simulink model "testfx"  (Simulink 6.0)
settings: Solver=ode45  StartTime=0.0  StopTime=10.0  RelTol=1e-3
InitFcn:
  | ;
StartFcn:
  | ;
StopFcn:
  | ;
undefined symbols (not defined in the file or in its folder): dden, tsamp
libraries: simulink x8
PreSaveFcn:
  | ;
CloseFcn:
  | rtwprivate ssgencode ModelCloseRequest testfx;
settings Model: Creator=myunt  LastModifiedBy=myunt  ExtModeAutoUpdateStatusClock=off
settings DebuggingCC: CheckExecutionContextPreStartOutputMsg=on  CheckExecutionContextRuntimeOutputMsg=on

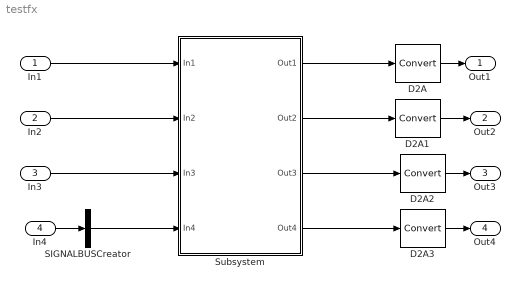
== system testfx ==
  In1 : Inport  LatchInput=off
  In2 : Inport  Port=2  LatchInput=off
  In3 : Inport  Port=3  LatchInput=off
  In4 : Inport  Port=4  LatchInput=off
  D2A{,1..3} (4 alike) : DataTypeConversion  OutDataTypeMode=double
  SIGNALBUSCreator : BusCreator  DialogController=Simulink.DDGSource_Bus  Inputs=1
  Subsystem : Subsystem  TreatAsAtomicUnit=on  PropExecContextAcrossSSBoundary=on
  Out1 : Outport
  Out2 : Outport  Port=2
  Out3 : Outport  Port=3
  Out4 : Outport  Port=4
  wires:
  In1/1 -> Subsystem/1(In1)
  Subsystem/1(Out1) -> D2A/1
  D2A/1 -> Out1/1
  Subsystem/2(Out2) -> D2A1/1
  D2A1/1 -> Out2/1
  In3/1 -> Subsystem/3(In3)
  Subsystem/3(Out3) -> D2A2/1
  D2A2/1 -> Out3/1
  Subsystem/4(Out4) -> D2A3/1
  D2A3/1 -> Out4/1
  In2/1 -> Subsystem/2(In2)
  In4/1 -> SIGNALBUSCreator/1
  SIGNALBUSCreator/1 -> Subsystem/4(In4)

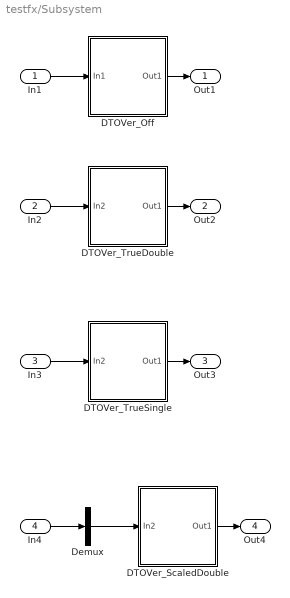
== system testfx/Subsystem ==
  In1 : Inport  LatchInput=off
  In2 : Inport  Port=2  LatchInput=off
  In3 : Inport  Port=3  LatchInput=off
  In4 : Inport  Port=4  LatchInput=off
  DTOVer_Off : Subsystem  PropExecContextAcrossSSBoundary=on
  DTOVer_ScaledDouble : Subsystem  PropExecContextAcrossSSBoundary=on  DataTypeOverride=ScaledDoubles
  DTOVer_TrueDouble : Subsystem  PropExecContextAcrossSSBoundary=on  DataTypeOverride=TrueDoubles
  DTOVer_TrueSingle : Subsystem  PropExecContextAcrossSSBoundary=on  DataTypeOverride=TrueSingles
  Demux : Demux  Outputs=1
  Out1 : Outport
  Out2 : Outport  Port=2
  Out3 : Outport  Port=3
  Out4 : Outport  Port=4
  wires:
  In1/1 -> DTOVer_Off/1(In1)
  DTOVer_Off/1(Out1) -> Out1/1
  In2/1 -> DTOVer_TrueDouble/1(In2)
  DTOVer_TrueDouble/1(Out1) -> Out2/1
  In3/1 -> DTOVer_TrueSingle/1(In2)
  DTOVer_TrueSingle/1(Out1) -> Out3/1
  In4/1 -> Demux/1
  Demux/1 -> DTOVer_ScaledDouble/1(In2)
  DTOVer_ScaledDouble/1(Out1) -> Out4/1

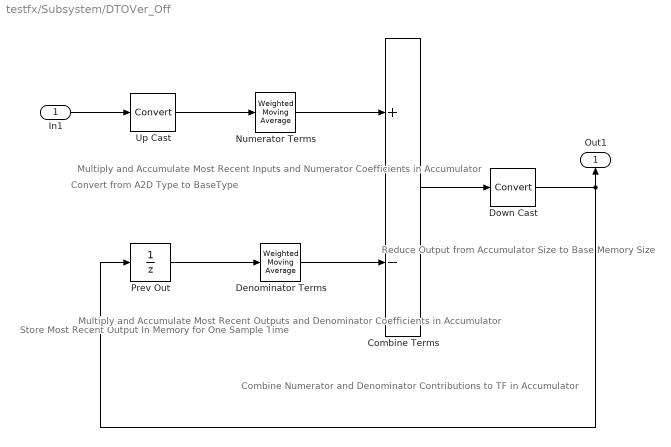
== system testfx/Subsystem/DTOVer_Off ==
  note: Reduce Output from
      | Accumulator Size to
      | Base Memory Size
  note: Combine Numerator
      | and Denominator
      | Contributions to TF
      | in Accumulator
  note: Store Most
      | Recent Output
      | In Memory for
      | One Sample Time
  note: Multiply and Accumulate
      | Most Recent Outputs and
      | Denominator Coefficients
      | in Accumulator
  note: Multiply and Accumulate
      | Most Recent Inputs and
      | Numerator Coefficients
      | in Accumulator
  note: Convert from
      | A2D Type
      | to BaseType
  In1 : Inport  DataType=Specify via dialog  OutScaling=2^-8  LatchInput=off
  Combine Terms : Sum  Inputs=+-  OutDataTypeMode=Specify via dialog  OutDataType=AccumType  OutScaling=2^(-12)  SaturateOnIntegerOverflow=on
  Denominator Terms : simulink/Discrete/Weighted Moving Average  mgainval=dden(2:length(dden))  vinit=0.0  samptime=tsamp  GainDataTypeScalingMode=Specify via dialog  GainDataType=BaseType  MatRadixGroup=Best Precision: Element-wise  GainScaling=2^-14  OutputDataTypeScalingMode=Specify via dialog  OutDataType=AccumType  OutScaling=2^(-12)  DoSatur=on
  Down Cast : DataTypeConversion  OutDataTypeMode=Specify via dialog  OutDataType=BaseType  OutScaling=2^(-5)  SaturateOnIntegerOverflow=on
  Numerator Terms : simulink/Discrete/Weighted Moving Average  mgainval=dnum  vinit=0.0  samptime=tsamp  GainDataTypeScalingMode=Specify via dialog  GainDataType=BaseType  MatRadixGroup=Best Precision: Element-wise  GainScaling=2^-14  OutputDataTypeScalingMode=Specify via dialog  OutDataType=AccumType  OutScaling=2^(-12)  DoSatur=on
  Prev Out : UnitDelay  X0=0.0  SampleTime=tsamp
  Up Cast : DataTypeConversion  OutDataTypeMode=Specify via dialog  OutDataType=BaseType  OutScaling=2^(-14)  SaturateOnIntegerOverflow=on
  Out1 : Outport  Orientation=up  InitialOutput=0
  wires:
  Down Cast/1 -> Out1/1, Prev Out/1
  In1/1 -> Up Cast/1
  Up Cast/1 -> Numerator Terms/1
  Prev Out/1 -> Denominator Terms/1
  Numerator Terms/1 -> Combine Terms/1
  Denominator Terms/1 -> Combine Terms/2
  Combine Terms/1 -> Down Cast/1

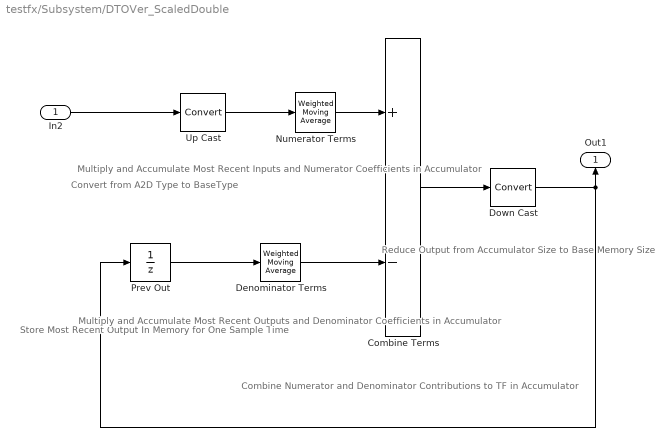
== system testfx/Subsystem/DTOVer_ScaledDouble ==
  note: Reduce Output from
      | Accumulator Size to
      | Base Memory Size
  note: Combine Numerator
      | and Denominator
      | Contributions to TF
      | in Accumulator
  note: Store Most
      | Recent Output
      | In Memory for
      | One Sample Time
  note: Multiply and Accumulate
      | Most Recent Outputs and
      | Denominator Coefficients
      | in Accumulator
  note: Multiply and Accumulate
      | Most Recent Inputs and
      | Numerator Coefficients
      | in Accumulator
  note: Convert from
      | A2D Type
      | to BaseType
  In2 : Inport  DataType=Specify via dialog  OutScaling=2^-8  LatchInput=off
  Combine Terms : Sum  Inputs=+-  OutDataTypeMode=Specify via dialog  OutDataType=AccumType  OutScaling=2^(-12)  SaturateOnIntegerOverflow=on
  Denominator Terms : simulink/Discrete/Weighted Moving Average  mgainval=dden(2:length(dden))  vinit=0.0  samptime=tsamp  GainDataTypeScalingMode=Specify via dialog  GainDataType=BaseType  MatRadixGroup=Best Precision: Element-wise  GainScaling=2^-14  OutputDataTypeScalingMode=Specify via dialog  OutDataType=AccumType  OutScaling=2^(-12)  DoSatur=on
  Down Cast : DataTypeConversion  OutDataTypeMode=Specify via dialog  OutDataType=BaseType  OutScaling=2^(-5)  SaturateOnIntegerOverflow=on
  Numerator Terms : simulink/Discrete/Weighted Moving Average  mgainval=dnum  vinit=0.0  samptime=tsamp  GainDataTypeScalingMode=Specify via dialog  GainDataType=BaseType  MatRadixGroup=Best Precision: Element-wise  GainScaling=2^-14  OutputDataTypeScalingMode=Specify via dialog  OutDataType=AccumType  OutScaling=2^(-12)  DoSatur=on
  Prev Out : UnitDelay  X0=0.0  SampleTime=tsamp
  Up Cast : DataTypeConversion  OutDataTypeMode=Specify via dialog  OutDataType=BaseType  OutScaling=2^(-14)  SaturateOnIntegerOverflow=on
  Out1 : Outport  Orientation=up  InitialOutput=0
  wires:
  Down Cast/1 -> Out1/1, Prev Out/1
  In2/1 -> Up Cast/1
  Up Cast/1 -> Numerator Terms/1
  Prev Out/1 -> Denominator Terms/1
  Numerator Terms/1 -> Combine Terms/1
  Denominator Terms/1 -> Combine Terms/2
  Combine Terms/1 -> Down Cast/1

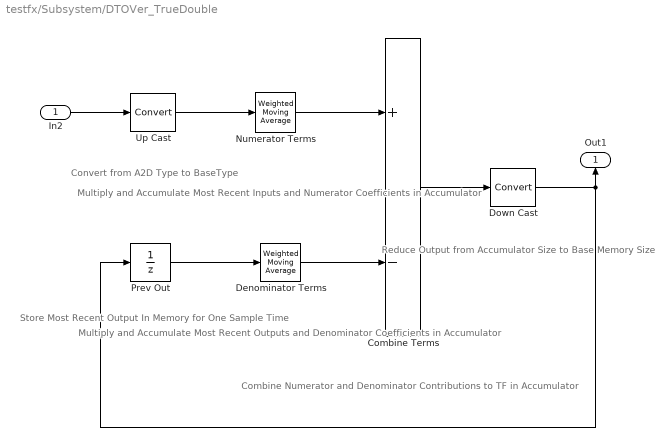
== system testfx/Subsystem/DTOVer_TrueDouble ==
  note: Convert from
      | A2D Type
      | to BaseType
  note: Multiply and Accumulate
      | Most Recent Inputs and
      | Numerator Coefficients
      | in Accumulator
  note: Multiply and Accumulate
      | Most Recent Outputs and
      | Denominator Coefficients
      | in Accumulator
  note: Store Most
      | Recent Output
      | In Memory for
      | One Sample Time
  note: Combine Numerator
      | and Denominator
      | Contributions to TF
      | in Accumulator
  note: Reduce Output from
      | Accumulator Size to
      | Base Memory Size
  In2 : Inport  DataType=Specify via dialog  OutScaling=2^-8  LatchInput=off
  Combine Terms : Sum  Inputs=+-  OutDataTypeMode=Specify via dialog  OutDataType=AccumType  OutScaling=2^(-12)  SaturateOnIntegerOverflow=on
  Denominator Terms : simulink/Discrete/Weighted Moving Average  mgainval=dden(2:length(dden))  vinit=0.0  samptime=tsamp  GainDataTypeScalingMode=Specify via dialog  GainDataType=BaseType  MatRadixGroup=Best Precision: Element-wise  GainScaling=2^-14  OutputDataTypeScalingMode=Specify via dialog  OutDataType=AccumType  OutScaling=2^(-12)  DoSatur=on
  Down Cast : DataTypeConversion  OutDataTypeMode=Specify via dialog  OutDataType=BaseType  OutScaling=2^(-5)  SaturateOnIntegerOverflow=on
  Numerator Terms : simulink/Discrete/Weighted Moving Average  mgainval=dnum  vinit=0.0  samptime=tsamp  GainDataTypeScalingMode=Specify via dialog  GainDataType=BaseType  MatRadixGroup=Best Precision: Element-wise  GainScaling=2^-14  OutputDataTypeScalingMode=Specify via dialog  OutDataType=AccumType  OutScaling=2^(-12)  DoSatur=on
  Prev Out : UnitDelay  X0=0.0  SampleTime=tsamp
  Up Cast : DataTypeConversion  OutDataTypeMode=Specify via dialog  OutDataType=BaseType  OutScaling=2^(-14)  SaturateOnIntegerOverflow=on
  Out1 : Outport  Orientation=up  InitialOutput=0
  wires:
  Combine Terms/1 -> Down Cast/1
  Denominator Terms/1 -> Combine Terms/2
  Numerator Terms/1 -> Combine Terms/1
  Prev Out/1 -> Denominator Terms/1
  Up Cast/1 -> Numerator Terms/1
  In2/1 -> Up Cast/1
  Down Cast/1 -> Prev Out/1, Out1/1

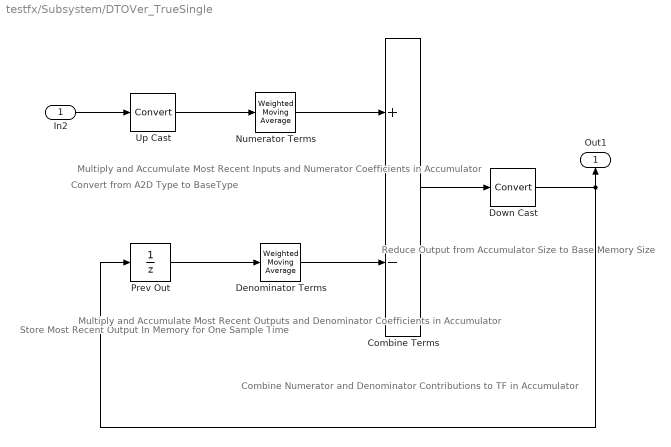
== system testfx/Subsystem/DTOVer_TrueSingle ==
  note: Reduce Output from
      | Accumulator Size to
      | Base Memory Size
  note: Combine Numerator
      | and Denominator
      | Contributions to TF
      | in Accumulator
  note: Store Most
      | Recent Output
      | In Memory for
      | One Sample Time
  note: Multiply and Accumulate
      | Most Recent Outputs and
      | Denominator Coefficients
      | in Accumulator
  note: Multiply and Accumulate
      | Most Recent Inputs and
      | Numerator Coefficients
      | in Accumulator
  note: Convert from
      | A2D Type
      | to BaseType
  In2 : Inport  DataType=Specify via dialog  OutScaling=2^-8  LatchInput=off
  Combine Terms : Sum  Inputs=+-  OutDataTypeMode=Specify via dialog  OutDataType=AccumType  OutScaling=2^(-12)  SaturateOnIntegerOverflow=on
  Denominator Terms : simulink/Discrete/Weighted Moving Average  mgainval=dden(2:length(dden))  vinit=0.0  samptime=tsamp  GainDataTypeScalingMode=Specify via dialog  GainDataType=BaseType  MatRadixGroup=Best Precision: Element-wise  GainScaling=2^-14  OutputDataTypeScalingMode=Specify via dialog  OutDataType=AccumType  OutScaling=2^(-12)  DoSatur=on
  Down Cast : DataTypeConversion  OutDataTypeMode=Specify via dialog  OutDataType=BaseType  OutScaling=2^(-5)  SaturateOnIntegerOverflow=on
  Numerator Terms : simulink/Discrete/Weighted Moving Average  mgainval=dnum  vinit=0.0  samptime=tsamp  GainDataTypeScalingMode=Specify via dialog  GainDataType=BaseType  MatRadixGroup=Best Precision: Element-wise  GainScaling=2^-14  OutputDataTypeScalingMode=Specify via dialog  OutDataType=AccumType  OutScaling=2^(-12)  DoSatur=on
  Prev Out : UnitDelay  X0=0.0  SampleTime=tsamp
  Up Cast : DataTypeConversion  OutDataTypeMode=Specify via dialog  OutDataType=BaseType  OutScaling=2^(-14)  SaturateOnIntegerOverflow=on
  Out1 : Outport  Orientation=up  InitialOutput=0
  wires:
  Down Cast/1 -> Out1/1, Prev Out/1
  In2/1 -> Up Cast/1
  Up Cast/1 -> Numerator Terms/1
  Prev Out/1 -> Denominator Terms/1
  Numerator Terms/1 -> Combine Terms/1
  Denominator Terms/1 -> Combine Terms/2
  Combine Terms/1 -> Down Cast/1
